simulink model "QuadModelv"  (R2022a)
settings: Solver=ode4  StartTime=0.0  StopTime=inf  FixedStep=0.001  RelTol=1e-3
PreLoadFcn:
  | filepath  = fileparts(get_param(bdroot, 'FileName'));
  | cd(filepath);
InitFcn:
  | Init
values from neighbouring files (symbols this model uses):
  ModelFailEnable = 0    [Init.m]
  ModelInit_RPM = 0    [Init.m]
  ModelParam_BattHoverMinutes = 18    [Init.m]
  ModelParam_BattHoverThr = 0.609    [Init.m]
  ModelParam_envAltitude = -50    [Init.m]
  ModelParam_GPSEphFinal = 0.3    [Init.m]
  ModelParam_GPSEpvFinal = 0.4    [Init.m]
  ModelParam_GPSFix3DFix = 3    [Init.m]
  ModelParam_GPSSatsVisible = 10    [Init.m]
  ModelParam_motorCr = 842.1    [Init.m]
  ModelParam_motorJm = 0.0001287    [Init.m]
  ModelParam_motorMinThr = 0.05    [Init.m]
  ModelParam_motorT = 0.0214    [Init.m]
  ModelParam_motorWb = 22.83    [Init.m]
  ModelParam_noiseGPSSampTime = 0.2    [Init.m]
  ModelParam_noisePowerOffGainAccel = 0.04    [Init.m]
  ModelParam_noisePowerOffGainAccelZ = 0.03    [Init.m]
  ModelParam_noisePowerOffGainGyro = 0.02    [Init.m]
  ModelParam_noisePowerOffGainGyroZ = 0.025    [Init.m]
  ModelParam_noisePowerOffGainMag = 0.02    [Init.m]
  ModelParam_noisePowerOffGainMagZ = 0.035    [Init.m]
  ModelParam_noisePowerOnGainAccel = 0.8    [Init.m]
  ModelParam_noisePowerOnGainAccelZ = 4.5    [Init.m]
  ModelParam_noisePowerOnGainGyro = 2    [Init.m]
  ModelParam_noisePowerOnGainGyroZ = 1    [Init.m]
  ModelParam_noisePowerOnGainMag = 0.025    [Init.m]
  ModelParam_noisePowerOnGainMagZ = 0.05    [Init.m]
  ModelParam_rotorCm = 2.783e-07    [Init.m]
  ModelParam_rotorCt = 1.681e-05    [Init.m]
  ModelParam_uavCCm = [0.0035 0.0039 0.0034]    [Init.m]
  ModelParam_uavCd = 0.055    [Init.m]
  ModelParam_uavDearo = 0.12    [Init.m]
  ModelParam_uavJ = [ModelParam_uavJxx,0,0;0,ModelParam_uavJyy,0;0,0,ModelParam_uavJzz]    [Init.m]
  ModelParam_uavMass = 1.515    [Init.m]
  ModelParam_uavMotNumbs = int8(4)    [Init.m]
  ModelParam_uavR = 0.225    [Init.m]
  ModelParam_uavType = int8(3)    [Init.m]
undefined symbols (not defined in the file or in its folder): d_i, Earth, h_i, ModelParam_GPSEpvInitial, ModelParam_GPSEpvTimeConstant, Newton, Raphson, WGS84
libraries: simulink x9, QuadModelLib x7, sharedtransform x3, aerolibtransform2 x2, sharedutil x2, aerolibutil x2, aerolibasang x2, shared6dof x1, aerolibatmos2 x1, aerolibconvert2 x1, aerolibobsolete x1
(part 1 of 3)
settings Model: Creator=Jinrui  LastModifiedBy=Tujinhu
settings SolverCC: AlgebraicLoopSolver=TrustRegion
settings DataIOCC: ReturnWorkspaceOutputs=off
settings OptimizationCC: ZeroExternalMemoryAtStartup=off  ZeroInternalMemoryAtStartup=off  EfficientTunableParamExpr=on
settings DebuggingCC: ParameterTunabilityLossMsg=error  UnconnectedInputMsg=warning  UnconnectedOutputMsg=warning  UnconnectedLineMsg=warning  SFMachineParentedDataDiag=warning  ArithmeticOperatorsInVariantConditions=warning
settings SFSimCC: SimUseLocalCustomCode=off  MATLABDynamicMemAlloc=off  CustomCodeUndefinedFunction=UseInterfaceOnly  SimTargetLang=C++
settings RTWCC: SystemTargetFile=ert.tlc  GenerateMakefile=off  PackageGeneratedCodeAndArtifacts=on  PackageName=MulticopterModel  TemplateMakefile=ert_default_tmf  RTWUseLocalCustomCode=off  TargetLang=C++  RTWCompilerOptimization=on  DLArmComputeVersion=19.05
settings CodeAppCC: ForceParamTrailComments=on  OperatorAnnotations=on  SimulinkDataObjDesc=on  SFDataObjDesc=on  MATLABFcnDesc=on  InsertBlockDesc=on  StateflowObjectComments=on  MATLABSourceComments=on
settings ERTTargetCC: TargetLangStandard=C++03 (ISO)  MultiwordLength=2048  GenerateSampleERTMain=on  CodeInterfacePackaging=C++ class  SupportContinuousTime=on  SupportVariableSizeSignals=on  MultiInstanceErrorCode=None  RootIOFormat=Structure reference  ERTCustomFileTemplate=example_file_process.tlc  ERTFilePackagingFormat=Compact
settings SimscapeCC: SimscapeNormalizeSystem=off

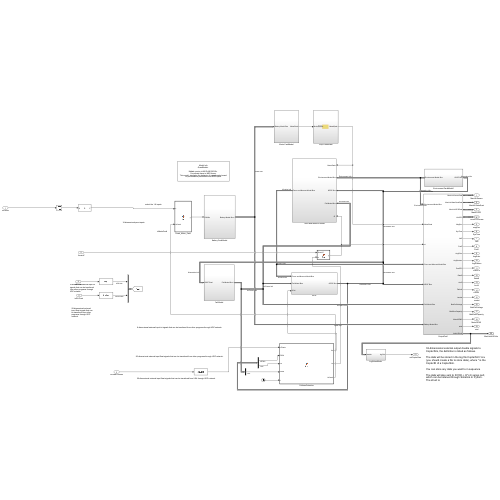
[thumbnail: Simulink's stored preview of the top-level diagram]
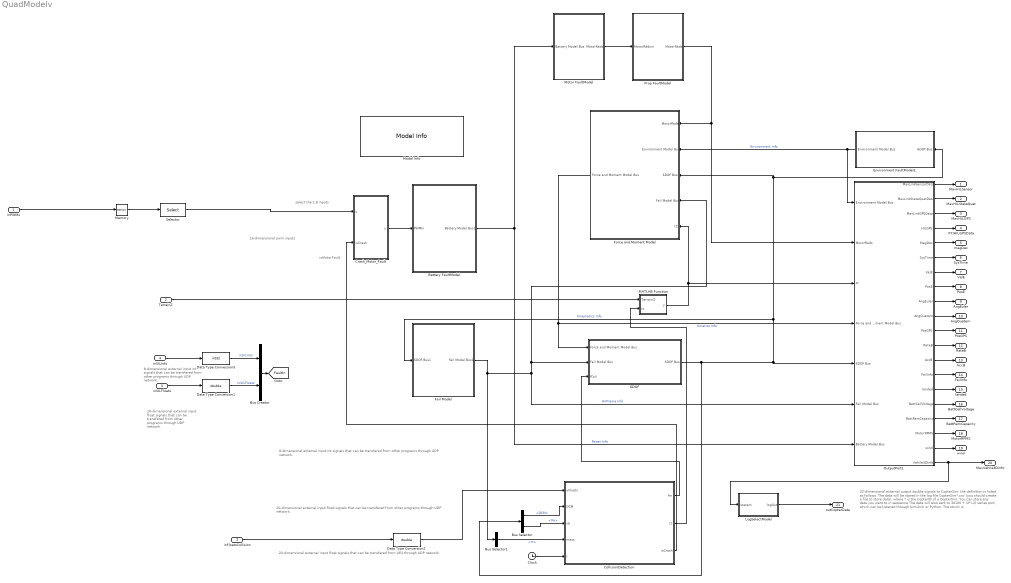
== system QuadModelv ==
  note: 16-dimensional pwm inputs
  note: 20-dimensional external input float signals that can be transfered from UE4 through UDP network.
  note: select the 1:8 inputs
  note: 8-dimensional external input int signals that can be transfered from other programs through UDP network.
  note: 20-dimensional external input float signals that can be transfered from other programs through UDP network.
  note: isMotorFault
  note: 20-dimensional external input float signals that can be transfered from other programs through UDP network.
  note: 8-dimensional external input int signals that can be transfered from other programs through UDP network.
  note: 32-dimensional external output double signals to CopterSim, the definition is listed as follows.
      |
      | The data will be stored in the log file CopterSim*.csv (you should create a file to store data), where * is the CopterID of a CopterSim.
      |
      | You can store any data you want to in sequence
      |
      | The data will also sent to 30100 + (2*i-2) series port, which can be listened through Simulink or Python. The struct is
  inPWMs : Inport  PortDimensions=8
  TerrainZ : Inport  Port=2  PortDimensions=1
  inFloatsCollision : Inport  Port=3  OutDataTypeStr=single  PortDimensions=20
  inSILInts : Inport  Port=4  OutDataTypeStr=int32  PortDimensions=8
  inSILFloats : Inport  Port=5  OutDataTypeStr=single  PortDimensions=20
  6DOF : Subsystem
  Battery FaultModel : Subsystem
  Bus Creator : BusCreator  Inputs=2
  Bus Selector : BusSelector  OutputSignals=DCM,Ve
  Bus Selector1 : BusSelector  OutputSignals=m
  Clock : Clock
  CollisionDetection : MATLAB Function  TreatAsAtomicUnit=on
  Crash_Motor_Fault : MATLAB Function  TreatAsAtomicUnit=on
  Data Type Conversion1 : DataTypeConversion  OutDataTypeStr=double  SaturateOnIntegerOverflow=off  RndMeth=Floor
  Data Type Conversion2 : DataTypeConversion  OutDataTypeStr=double  SaturateOnIntegerOverflow=off  RndMeth=Floor
  Data Type Conversion3 : DataTypeConversion  OutDataTypeStr=int32  SaturateOnIntegerOverflow=off  RndMeth=Floor
  Environment FaultModel1 : Subsystem
  Fail Model : Subsystem
  Force and Moment Model : Subsystem
  LogSelectModel : Subsystem
  MATLAB Function : MATLAB Function  TreatAsAtomicUnit=on
  Memory : Memory
  Model Info : simulink/Model-Wide Utilities/Model Info  Frame=on  DisplayStringWithTags=|  HorizontalTextAlignment=Center  LeftAlignmentValue=0.5
      | Model Info
      | %<ModelName> 
      | %<Description>   
      | Matlab version is MATLAB R2016b. 
      | Coordinate frame is NED frame.
      |  This model  simulates the behavior of a quadcopter based 
      | on performance parameters and RPM inputs
  Motor FaultModel : Subsystem
  OutputPort1 : Subsystem
  Prop FaultModel : Subsystem
  Selector : Selector  InputPortWidth=8  IndexOptions=Index vector (dialog)  Indices=[1:8]  OutputSizes=1
  MavHILSensor : Outport
  MavHILStateQuat : Outport  Port=2  OutDataTypeStr=Bus: MavLinkStateQuat  VectorParamsAs1DForOutWhenUnconnected=off
  MavHILGPS : Outport  Port=3
  PXIHILGPSData : Outport  Port=4  OutDataTypeStr=Bus: HILGPS  VectorParamsAs1DForOutWhenUnconnected=off
  magDec : Outport  Port=5  VectorParamsAs1DForOutWhenUnconnected=off
  SysTime : Outport  Port=6  VectorParamsAs1DForOutWhenUnconnected=off
  VelE : Outport  Port=7  VectorParamsAs1DForOutWhenUnconnected=off
  PosE : Outport  Port=8  VectorParamsAs1DForOutWhenUnconnected=off
  AngEuler : Outport  Port=9  VectorParamsAs1DForOutWhenUnconnected=off
  AngQuatern : Outport  Port=10  VectorParamsAs1DForOutWhenUnconnected=off
  PosGPS : Outport  Port=11  VectorParamsAs1DForOutWhenUnconnected=off
  RateB : Outport  Port=12  VectorParamsAs1DForOutWhenUnconnected=off
  AccB : Outport  Port=13  VectorParamsAs1DForOutWhenUnconnected=off
  FailInfo : Outport  Port=14  VectorParamsAs1DForOutWhenUnconnected=off
  landed : Outport  Port=15  VectorParamsAs1DForOutWhenUnconnected=off
  BattCellVoltage : Outport  Port=16  VectorParamsAs1DForOutWhenUnconnected=off
  BattRemCapacity : Outport  Port=17  VectorParamsAs1DForOutWhenUnconnected=off
  MotorRPMS : Outport  Port=18  VectorParamsAs1DForOutWhenUnconnected=off
  wind : Outport  Port=19  VectorParamsAs1DForOutWhenUnconnected=off
  MavVehile3DInfo : Outport  Port=20  OutDataTypeStr=Bus: MavVehileInfo  VectorParamsAs1DForOutWhenUnconnected=off
  outCopterData : Outport  Port=21  OutDataTypeStr=double  PortDimensions=32  VectorParamsAs1DForOutWhenUnconnected=off
  tag scope: FaultIn=global
  wires:
  OutputPort1/14(FailInfo) -> FailInfo/1
  OutputPort1/9(AngEuler) -> AngEuler/1
  OutputPort1/17(BattRemCapacity) -> BattRemCapacity/1
  Memory/1 -> Selector/1
  OutputPort1/1(MavLinkSensorData) -> MavHILSensor/1
  Force and Moment Model/1(Force and Moment Model Bus) -> 6DOF/1(Force and Moment Model Bus), OutputPort1/4(Force and Moment Model Bus)  "Kinetics Info"
  Battery FaultModel/1(Battery Model Bus1) -> Motor FaultModel/1(Battery Model Bus), OutputPort1/7(Battery Model Bus)  "Power Info"
  Fail Model/1(Fail Model Bus1) -> Bus Selector1/1, Force and Moment Model/4(Fail Model Bus), 6DOF/2(Fail Model Bus), OutputPort1/6(Fail Model Bus)  "AirFrame Info"
  Bus Selector1/1 -> CollisionDetection/4(mass)  "<m>"
  OutputPort1/15(landed) -> landed/1
  TerrainZ/1 -> MATLAB Function/1(TerrainZ)
  OutputPort1/8(PosE) -> PosE/1
  OutputPort1/19(wind) -> wind/1
  Environment FaultModel1/1(Environment Model Bus) -> OutputPort1/1(Environment Model Bus), Force and Moment Model/2(Environment Model Bus)  "Environment Info"
  inFloatsCollision/1 -> Data Type Conversion2/1
  Bus Selector/1 -> CollisionDetection/2(DCM)  "<DCM>"
  inPWMs/1 -> Memory/1
  MATLAB Function/1(y) -> Force and Moment Model/5("tZ "), OutputPort1/3(zt)
  CollisionDetection/2(tz) -> MATLAB Function/2(tz)
  Prop FaultModel/1(MotorRads) -> OutputPort1/2(MotorRads), Force and Moment Model/1(MotorRads)
  OutputPort1/10(AngQuatern) -> AngQuatern/1
  OutputPort1/7(VelE) -> VelE/1
  OutputPort1/13(AccB) -> AccB/1
  6DOF/1(6DOF Bus) -> Bus Selector/1, Fail Model/1(6DOF Bus1), Environment FaultModel1/1(6DOF Bus), Force and Moment Model/3(6DOF Bus), OutputPort1/5(6DOF Bus)  "Kinematics Info"
  OutputPort1/12(RateB) -> RateB/1
  OutputPort1/5(MagDec) -> magDec/1
  CollisionDetection/1(fm) -> 6DOF/3(fColi)
  OutputPort1/18(MotorRPMS) -> MotorRPMS/1
  OutputPort1/16(BattCellVoltage) -> BattCellVoltage/1
  OutputPort1/20(Vehile3DInfo) -> LogSelectModel/1(stateIn), MavVehile3DInfo/1
  CollisionDetection/3(isCrash) -> Crash_Motor_Fault/2(isCrash)
  Bus Selector/2 -> CollisionDetection/3(ve)  "<Ve>"
  OutputPort1/2(MavLinkStateQuatData) -> MavHILStateQuat/1
  OutputPort1/3(MavLinkGPSData) -> MavHILGPS/1
  Data Type Conversion2/1 -> CollisionDetection/1(uFloats)
  OutputPort1/6(SysTime) -> SysTime/1
  OutputPort1/4(HILGPS) -> PXIHILGPSData/1
  OutputPort1/11(PosGPS) -> PosGPS/1
  Clock/1 -> CollisionDetection/5(t)
  Data Type Conversion3/1 -> Bus Creator/1  "inSILInts"
  Data Type Conversion1/1 -> Bus Creator/2  "inSILFloats"
  Bus Creator/1 -> [FaultIn]
  LogSelectModel/1(logOut) -> outCopterData/1
  Motor FaultModel/1(MotorRads) -> Prop FaultModel/1(MotorRadsin)
  Crash_Motor_Fault/1(y) -> Battery FaultModel/1(PWMIn)
  Selector/1 -> Crash_Motor_Fault/1(u)
  inSILInts/1 -> Data Type Conversion3/1
  inSILFloats/1 -> Data Type Conversion1/1

== system QuadModelv/6DOF ==
  Force and Moment Model Bus : Inport
  Fail Model Bus : Inport  Port=2
  fColi : Inport  Port=3
  Bus Creator : BusCreator  Inputs=8
  Bus Selector : BusSelector  OutputSignals=dM,m,J
  Bus Selector1 : BusSelector  OutputSignals=Fb,Mb
  Constant_dI/dt : Constant  Value=zeros(3,3)
  Custom Variable Mass 6DOF (Quaternion) : shared6dof/6DOF (Euler Angles)  units=Metric (MKS)  mtype=Custom Variable  rep=Quaternion  xme_0=ModelInit_PosE  Vm_0=ModelInit_VelB  eul_0=ModelInit_AngEuler  pm_0=ModelInit_RateB  mass_0=1.0  mass_e=0.5  mass_f=2.0  inertia=eye(3)  inertia_e=eye(3)  inertia_f=2*eye(3)  k_quat=1.0  vre_flag=off  abi_flag=off  aMode=aMode  xme_statename=''  Vm_statename=''  eul_statename=''  quat_statename=''  pm_statename=''  mass_statename=''
      settings: SourceProductBaseCode=AE,PW,DR,MT,VE
  Demux : Demux  Outputs=2
  Sum : Sum  Inputs=+++
  Sum1 : Sum  Inputs=++|
  6DOF Bus : Outport  VectorParamsAs1DForOutWhenUnconnected=off
  wires:
  Bus Selector1/1 -> Sum1/2  "<Fb>"
  Bus Selector/2 -> Custom Variable Mass 6DOF (Quaternion)/3  "<m>"
  Custom Variable Mass 6DOF (Quaternion)/8 -> Bus Creator/8  "AccB"
  Sum/1 -> Custom Variable Mass 6DOF (Quaternion)/2
  Constant_dI/dt/1 -> Custom Variable Mass 6DOF (Quaternion)/4
  Custom Variable Mass 6DOF (Quaternion)/5 -> Bus Creator/5  "Vb"
  Custom Variable Mass 6DOF (Quaternion)/6 -> Bus Creator/6  "wb"
  Custom Variable Mass 6DOF (Quaternion)/1 -> Bus Creator/1  "Ve"
  Custom Variable Mass 6DOF (Quaternion)/4 -> Bus Creator/4  "DCM"
  Custom Variable Mass 6DOF (Quaternion)/2 -> Bus Creator/2  "Xe"
  Custom Variable Mass 6DOF (Quaternion)/3 -> Bus Creator/3  "Eular(rad)"
  Custom Variable Mass 6DOF (Quaternion)/7 -> Bus Creator/7  "dwb/dt"
  Bus Selector/3 -> Custom Variable Mass 6DOF (Quaternion)/5  "<J>"
  Bus Selector/1 -> Sum/2  "<dM>"
  Bus Selector1/2 -> Sum/1  "<Mb>"
  Fail Model Bus/1 -> Bus Selector/1
  Force and Moment Model Bus/1 -> Bus Selector1/1
  Bus Creator/1 -> 6DOF Bus/1
  Sum1/1 -> Custom Variable Mass 6DOF (Quaternion)/1
  Demux/1 -> Sum1/1
  fColi/1 -> Demux/1
  Demux/2 -> Sum/3

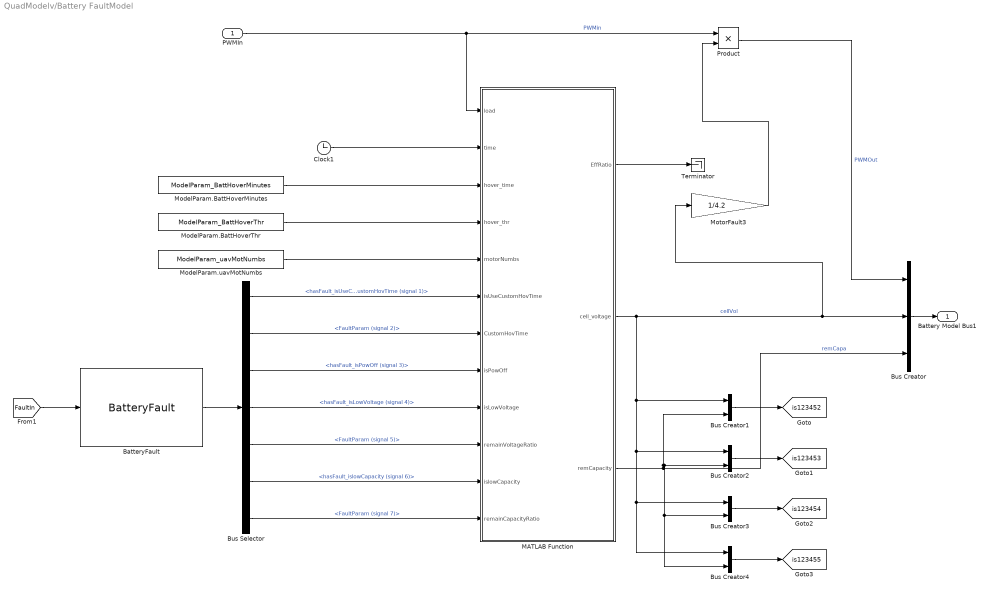
== system QuadModelv/Battery FaultModel ==
  PWMIn : Inport
  BatteryFault : QuadModelLib/BatteryFault  FaultParamStruct=BatteryFault
  Bus Creator : BusCreator  Inputs=3
  Bus Creator{1..4} (4 alike) : BusCreator  Inputs=2
  Bus Selector : BusSelector  OutputSignals=hasFault_isUseCustomHovTime (signal 1),FaultParam (signal 2),hasFault_isPowOff (signal 3),hasFault_isLowVoltage (signal 4),FaultParam (signal 5),hasFault_islowCapacity (signal 6),FaultParam (signal 7)
  Clock1 : Clock
  MATLAB Function : MATLAB Function  TreatAsAtomicUnit=on  SystemSampleTime=0.01
  ModelParam.BattHoverMinutes : Constant  Value=ModelParam_BattHoverMinutes
  ModelParam.BattHoverThr : Constant  Value=ModelParam_BattHoverThr
  ModelParam.uavMotNumbs : Constant  Value=ModelParam_uavMotNumbs
  MotorFault3 : Gain  Gain=1/4.2
  Product : Product
  Terminator : Terminator
  Battery Model Bus1 : Outport  VectorParamsAs1DForOutWhenUnconnected=off
  tag scope: is123452=global, is123453=global, is123454=global, is123455=global
  wires:
  Bus Selector/7 -> MATLAB Function/12(remainCapacityRatio)  "<FaultParam (signal 7)>"
  Bus Creator4/1 -> [is123455]
  MATLAB Function/2(cell_voltage) -> Bus Creator4/1, Bus Creator3/1, Bus Creator2/1, Bus Creator1/1, MotorFault3/1, Bus Creator/2  "cellVol"
  MATLAB Function/3(remCapacity) -> Bus Creator1/2, Bus Creator4/2, Bus Creator3/2, Bus Creator2/2, Bus Creator/3  "remCapa"
  Bus Selector/2 -> MATLAB Function/7(CustomHovTime)  "<FaultParam (signal 2)>"
  ModelParam.uavMotNumbs/1 -> MATLAB Function/5(motorNumbs)
  Bus Creator/1 -> Battery Model Bus1/1
  Bus Creator1/1 -> [is123452]
  Bus Creator2/1 -> [is123453]
  ModelParam.BattHoverThr/1 -> MATLAB Function/4(hover_thr)
  Bus Creator3/1 -> [is123454]
  MATLAB Function/1(EffRatio) -> Terminator/1
  ModelParam.BattHoverMinutes/1 -> MATLAB Function/3(hover_time)
  Product/1 -> Bus Creator/1  "PWMOut"
  PWMIn/1 -> MATLAB Function/1(load), Product/1  "PWMin"
  Bus Selector/6 -> MATLAB Function/11(islowCapacity)  "<hasFault_islowCapacity (signal 6)>"
  Bus Selector/3 -> MATLAB Function/8(isPowOff)  "<hasFault_isPowOff (signal 3)>"
  Clock1/1 -> MATLAB Function/2(time)
  BatteryFault/1 -> Bus Selector/1
  Bus Selector/4 -> MATLAB Function/9(isLowVoltage)  "<hasFault_isLowVoltage (signal 4)>"
  [FaultIn] -> BatteryFault/1
  MotorFault3/1 -> Product/2
  Bus Selector/1 -> MATLAB Function/6(isUseCustomHovTime)  "<hasFault_isUseCustomHovTime (signal 1)>"
  Bus Selector/5 -> MATLAB Function/10(remainVoltageRatio)  "<FaultParam (signal 5)>"

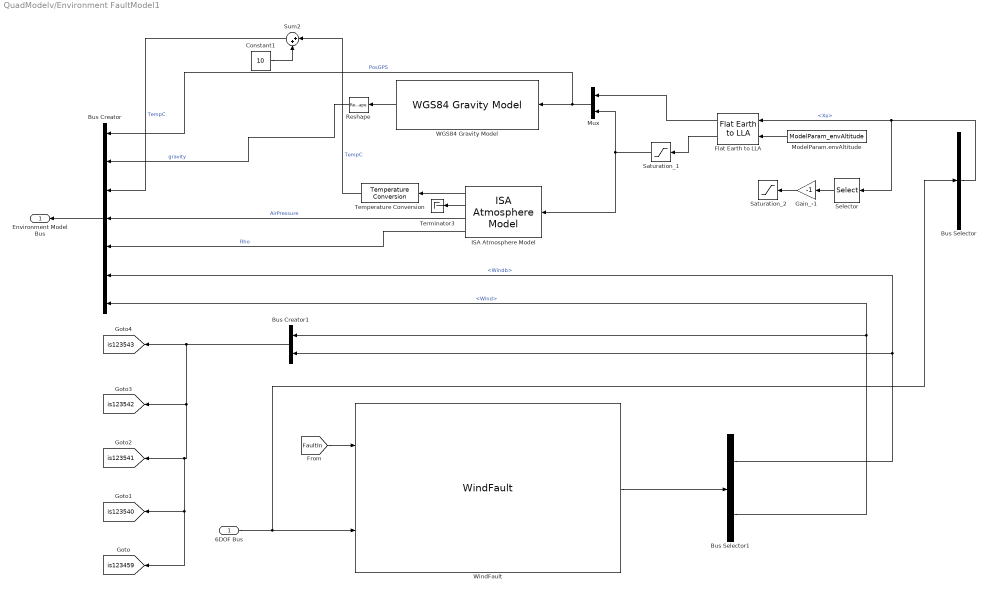
== system QuadModelv/Environment FaultModel1 ==
  6DOF Bus : Inport
  Bus Creator : BusCreator  Inputs=7
  Bus Creator1 : BusCreator  Inputs=2
  Bus Selector : BusSelector  OutputSignals=Xe
  Bus Selector1 : BusSelector  OutputSignals=Windb,Wind
  Constant1 : Constant  Value=10
  Flat Earth to LLA : aerolibtransform2/Flat Earth to LLA  units=Metric (MKS)  ptype=Earth (WGS84)  F=1/298.257223563  R=6378137  refPosPort=off  LL0=ModelParam_GPSLatLong  psi=0
  Gain_-1 : Gain  Gain=-1
  ISA Atmosphere Model : aerolibatmos2/ISA Atmosphere Model  custom=off  g=9.80665  gamma=1.4  R=287.0531  L=0.0065  h_trop=11000  h_strat=20000  rho0=1.225  P0=101325  T0=288.15  h0=0
  ModelParam.envAltitude : Constant  Value=ModelParam_envAltitude
  Mux : Mux  Inputs=2
  Reshape : Reshape
  Saturation_1 : Saturate  UpperLimit=100000  LowerLimit=0
  Saturation_2 : Saturate  UpperLimit=10000  LowerLimit=0
  Selector : Selector  InputPortWidth=3  IndexOptions=Index vector (dialog)  Indices=[3]  OutputSizes=1
  Sum2 : Sum  Inputs=|++
  Temperature Conversion : aerolibconvert2/Temperature Conversion  IU=K  OU=C
      settings: SourceProductBaseCode=AE
  Terminator3 : Terminator
  "WGS84 Gravity Model " : aerolibobsolete/WGS84 Gravity Model   model=WGS84 Taylor Series  units=Metric (MKS)  no_atmos=on  precessing=on  jd_loc=off  month=October  day=10  year=2004  no_centrifugal=on  action=Warning
      settings: SourceProductBaseCode=AE
  WindFault : QuadModelLib/WindFault  FaultParamStruct=WindFault  ComParamVect=FaultParamAPI
  Environment Model Bus : Outport  VectorParamsAs1DForOutWhenUnconnected=off
  tag scope: is123459=global, is123540=global, is123541=global, is123542=global, is123543=global
  wires:
  ISA Atmosphere Model/2 -> Terminator3/1
  Bus Selector/1 -> Selector/1, Flat Earth to LLA/1  "<Xe>"
  Flat Earth to LLA/1 -> Mux/1
  Mux/1 -> Bus Creator/1, "WGS84 Gravity Model "/1  "PosGPS"
  ISA Atmosphere Model/3 -> Bus Creator/4  "AirPressure"
  Selector/1 -> Gain_-1/1
  Sum2/1 -> Bus Creator/3  "TempC"
  Temperature Conversion/1 -> Sum2/1  "TempC"
  ModelParam.envAltitude/1 -> Flat Earth to LLA/2
  Constant1/1 -> Sum2/2
  Reshape/1 -> Bus Creator/2  "gravity"
  "WGS84 Gravity Model "/1 -> Reshape/1
  Gain_-1/1 -> Saturation_2/1
  6DOF Bus/1 -> WindFault/2, Bus Selector/1
  Bus Creator/1 -> Environment Model Bus/1
  Bus Selector1/2 -> Bus Creator/7, Bus Creator1/1  "<Wind>"
  Bus Creator1/1 -> [is123459], [is123540], [is123541], [is123542], [is123543]
  ISA Atmosphere Model/1 -> Temperature Conversion/1
  Saturation_1/1 -> Mux/2, ISA Atmosphere Model/1
  Bus Selector1/1 -> Bus Creator/6, Bus Creator1/2  "<Windb>"
  [FaultIn] -> WindFault/1
  ISA Atmosphere Model/4 -> Bus Creator/5  "Rho"
  Flat Earth to LLA/2 -> Saturation_1/1
  WindFault/1 -> Bus Selector1/1

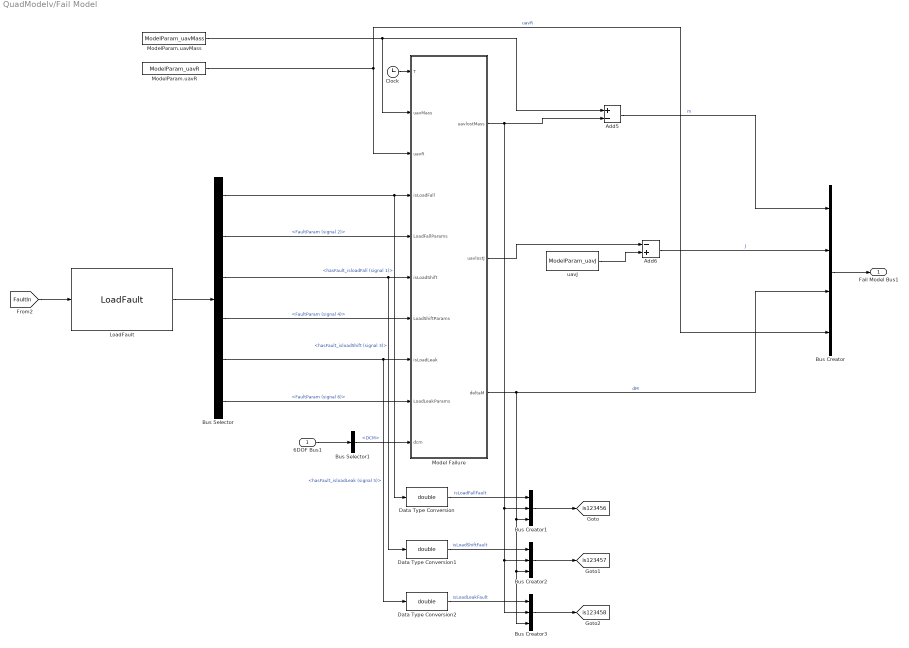
== system QuadModelv/Fail Model ==
  6DOF Bus1 : Inport
  Add5 : Sum  Inputs=+-
  Add6 : Sum  Inputs=-+
  Bus Creator : BusCreator  Inputs=4
  Bus Creator1 : BusCreator  Inputs=3
  Bus Creator2 : BusCreator  Inputs=3
  Bus Creator3 : BusCreator  Inputs=3
  Bus Selector : BusSelector  OutputSignals=hasFault_isloadFall (signal 1),FaultParam (signal 2),hasFault_isloadShift (signal 3),FaultParam (signal 4),hasFault_isloadLeak (signal 5),FaultParam (signal 6)
  Bus Selector1 : BusSelector  OutputSignals=DCM
  Clock : Clock
  Data Type Conversion : DataTypeConversion  OutDataTypeStr=double  SaturateOnIntegerOverflow=off  RndMeth=Floor
  Data Type Conversion1 : DataTypeConversion  OutDataTypeStr=double  SaturateOnIntegerOverflow=off  RndMeth=Floor
  Data Type Conversion2 : DataTypeConversion  OutDataTypeStr=double  SaturateOnIntegerOverflow=off  RndMeth=Floor
  LoadFault : QuadModelLib/LoadFault  FaultParamStruct=LoadFault
  Model Failure : MATLAB Function  TreatAsAtomicUnit=on
  ModelParam.uavMass : Constant  Value=ModelParam_uavMass
  ModelParam.uavR : Constant  Value=ModelParam_uavR
  uavJ : Constant  Value=ModelParam_uavJ
  Fail Model Bus1 : Outport  VectorParamsAs1DForOutWhenUnconnected=off
  tag scope: is123456=global, is123457=global, is123458=global
  wires:
  Bus Selector/3 -> Data Type Conversion1/1, Model Failure/6(isLoadShift)  "<hasFault_isloadShift (signal 3)>"
  Data Type Conversion2/1 -> Bus Creator3/1  "isLoadLeakFault"
  Model Failure/3(deltaM) -> Bus Creator1/3, Bus Creator3/3, Bus Creator2/3, Bus Creator/3  "dM"
  Data Type Conversion/1 -> Bus Creator1/1  "isLoadFallFault"
  Bus Creator2/1 -> [is123457]
  Bus Creator1/1 -> [is123456]
  Data Type Conversion1/1 -> Bus Creator2/1  "isLoadShiftFault"
  Bus Creator/1 -> Fail Model Bus1/1
  Bus Selector/6 -> Model Failure/9(LoadLeakParams)  "<FaultParam (signal 6)>"
  Bus Creator3/1 -> [is123458]
  Bus Selector1/1 -> Model Failure/10(dcm)  "<DCM>"
  uavJ/1 -> Add6/2
  Model Failure/2(uavlostJ) -> Add6/1
  ModelParam.uavR/1 -> Model Failure/3(uavR), Bus Creator/4  "uavR"
  Bus Selector/1 -> Model Failure/4(isLoadFall), Data Type Conversion/1  "<hasFault_isloadFall (signal 1)>"
  Add6/1 -> Bus Creator/2  "J"
  6DOF Bus1/1 -> Bus Selector1/1
  Bus Selector/2 -> Model Failure/5(LoadFallParams)  "<FaultParam (signal 2)>"
  Add5/1 -> Bus Creator/1  "m"
  Bus Selector/4 -> Model Failure/7(LoadShiftParams)  "<FaultParam (signal 4)>"
  Bus Selector/5 -> Data Type Conversion2/1, Model Failure/8(isLoadLeak)  "<hasFault_isloadLeak (signal 5)>"
  Clock/1 -> Model Failure/1(T)
  Model Failure/1(uavlostMass) -> Bus Creator1/2, Bus Creator3/2, Bus Creator2/2, Add5/2
  [FaultIn] -> LoadFault/1
  LoadFault/1 -> Bus Selector/1
  ModelParam.uavMass/1 -> Model Failure/2(uavMass), Add5/1

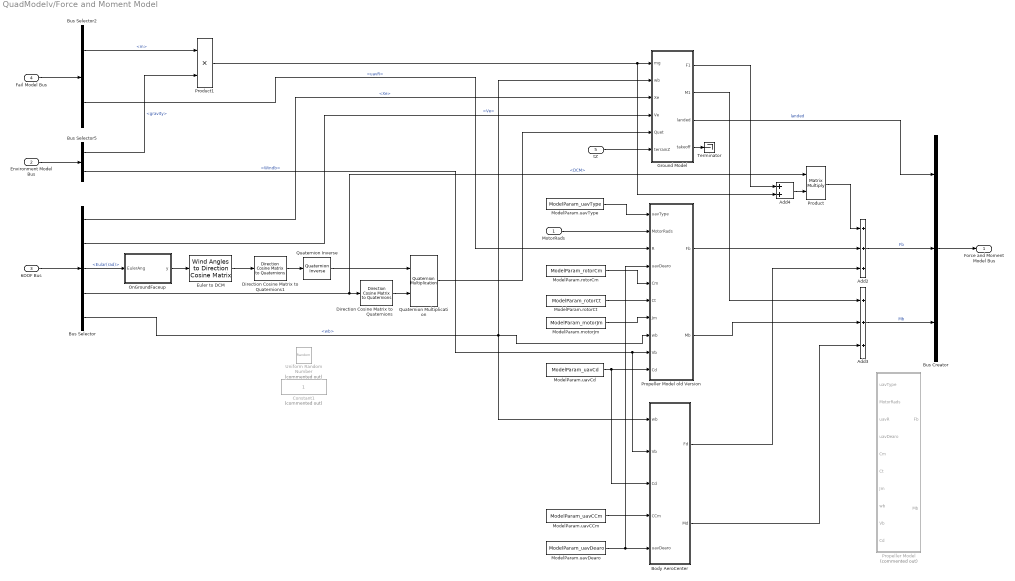
== system QuadModelv/Force and Moment Model ==
  MotorRads : Inport
  Environment Model Bus : Inport  Port=2
  6DOF Bus : Inport  Port=3
  Fail Model Bus : Inport  Port=4
  "tZ " : Inport  Port=5
  Add2 : Sum  Inputs=+++
  Add3 : Sum  Inputs=+++
  Add4 : Sum
  Body AeroCenter : MATLAB Function  TreatAsAtomicUnit=on
  Bus Creator : BusCreator  Inputs=3
  Bus Selector : BusSelector  OutputSignals=Xe,Ve,Eular(rad),DCM,wb
  Bus Selector2 : BusSelector  OutputSignals=m,uavR
  Bus Selector5 : BusSelector  OutputSignals=gravity,Windb
  Constant1 : Constant  Commented=on
  Direction Cosine Matrix to Quaternions : sharedtransform/Direction Cosine Matrix  to Quaternions  aMode=aMode  action=None  tolerance=eps(2)
      settings: SourceProductBaseCode=AE,PW,DR,MT,VE
  Direction Cosine Matrix to Quaternions1 : sharedtransform/Direction Cosine Matrix  to Quaternions  aMode=aMode  action=None  tolerance=eps(2)
      settings: SourceProductBaseCode=AE,PW,DR,MT,VE
  Euler to DCM : aerolibtransform2/Wind Angles to  Direction Cosine Matrix
      settings: SourceProductBaseCode=AE
  Ground Model : MATLAB Function  TreatAsAtomicUnit=on
  ModelParam.motorJm : Constant  Value=ModelParam_motorJm
  ModelParam.rotorCm : Constant  Value=ModelParam_rotorCm
  ModelParam.rotorCt : Constant  Value=ModelParam_rotorCt
  ModelParam.uavCCm : Constant  Value=ModelParam_uavCCm
  ModelParam.uavCd : Constant  Value=ModelParam_uavCd
  ModelParam.uavDearo : Constant  Value=ModelParam_uavDearo
  ModelParam.uavType : Constant  Value=ModelParam_uavType
  OnGroundFaceup : MATLAB Function  TreatAsAtomicUnit=on
  Product : Product  Multiplication=Matrix(*)
  Product1 : Product
  Propeller Model : Subsystem  Commented=on  TreatAsAtomicUnit=on
  Propeller Model old Version : MATLAB Function  TreatAsAtomicUnit=on
  Quaternion Inverse : aerolibutil/Quaternion Inverse
  Quaternion Multiplication : aerolibutil/Quaternion Multiplication
  Terminator : Terminator
  Uniform Random Number : UniformRandomNumber  Commented=on  Minimum=[-1,-1,-1]  Maximum=[1,1,1]  Seed=[145787,351545,2864]  SampleTime=0.05
  Force and Moment Model Bus : Outport  VectorParamsAs1DForOutWhenUnconnected=off
  wires:
  Body AeroCenter/2(Md) -> Add3/3
  Body AeroCenter/1(Fd) -> Add2/3
  Propeller Model old Version/2(Mb) -> Add3/2
  Propeller Model old Version/1(Fb) -> Add2/2
  Ground Model/4(takeoff) -> Terminator/1
  Ground Model/3(landed) -> Bus Creator/1  "landed"
  "tZ "/1 -> Ground Model/6(terrainZ)
  Add3/1 -> Bus Creator/3  "Mb"
  Add2/1 -> Bus Creator/2  "Fb"
  ModelParam.uavType/1 -> Propeller Model old Version/1(uavType)
  Quaternion Multiplication/1 -> Ground Model/5(Quet)
  Quaternion Inverse/1 -> Quaternion Multiplication/1
  Direction Cosine Matrix to Quaternions1/1 -> Quaternion Inverse/1
  Euler to DCM/1 -> Direction Cosine Matrix to Quaternions1/1
  OnGroundFaceup/1(y) -> Euler to DCM/1
  Direction Cosine Matrix to Quaternions/1 -> Quaternion Multiplication/2
  ModelParam.rotorCt/1 -> Propeller Model old Version/6(Ct)
  Product/1 -> Add2/1
  Ground Model/1(F1) -> Add4/1
  Add4/1 -> Product/2
  Product1/1 -> Ground Model/1(mg), Add4/2
  Ground Model/2(M1) -> Add3/1
  Bus Selector/4 -> Direction Cosine Matrix to Quaternions/1, Product/1  "<DCM>"
  ModelParam.uavCd/1 -> Body AeroCenter/3(Cd), Propeller Model old Version/10(Cd)
  ModelParam.motorJm/1 -> Propeller Model old Version/7(Jm)
  ModelParam.rotorCm/1 -> Propeller Model old Version/5(Cm)
  MotorRads/1 -> Propeller Model old Version/2(MotorRads)
  Bus Selector/5 -> Ground Model/2(wb), Propeller Model old Version/8(wb), Body AeroCenter/1(wb)  "<wb>"
  ModelParam.uavCCm/1 -> Body AeroCenter/4(CCm)
  Bus Creator/1 -> Force and Moment Model Bus/1
  6DOF Bus/1 -> Bus Selector/1
  Bus Selector/2 -> Ground Model/4(Ve)  "<Ve>"
  Bus Selector/1 -> Ground Model/3(Xe)  "<Xe>"
  Bus Selector/3 -> OnGroundFaceup/1(EulerAng)  "<Eular(rad)>"
  Bus Selector2/1 -> Product1/1  "<m>"
  Bus Selector5/1 -> Product1/2  "<gravity>"
  Fail Model Bus/1 -> Bus Selector2/1
  Environment Model Bus/1 -> Bus Selector5/1
  Bus Selector2/2 -> Propeller Model old Version/3(R)  "<uavR>"
  Bus Selector5/2 -> Body AeroCenter/2(Vb), Propeller Model old Version/9(Vb)  "<Windb>"
  ModelParam.uavDearo/1 -> Propeller Model old Version/4(uavDearo), Body AeroCenter/5(uavDearo)

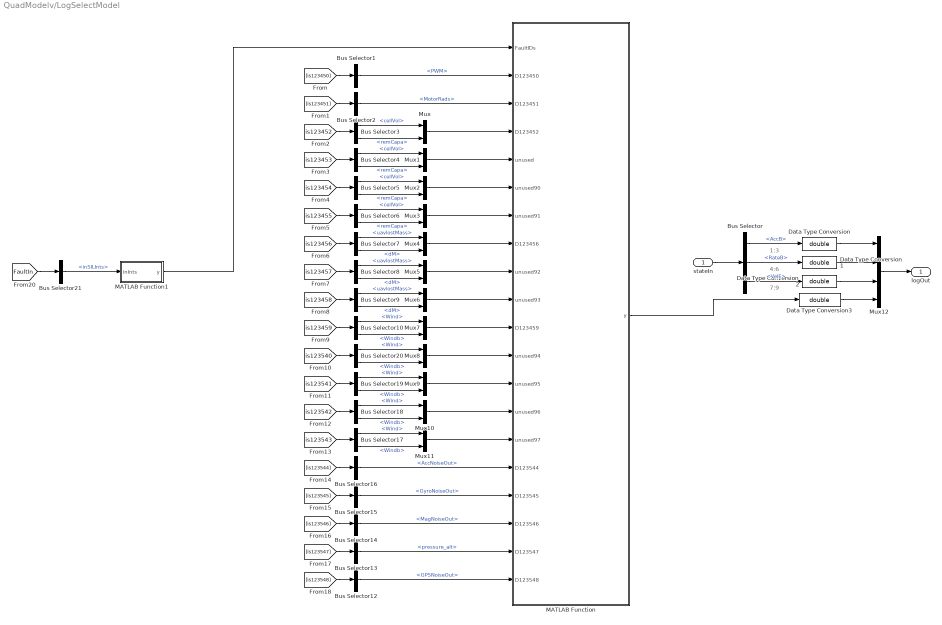
== system QuadModelv/LogSelectModel ==
  note: 1:3
  note: 4:6
  note: 7:9
  stateIn : Inport
  Bus Selector : BusSelector  OutputSignals=AccB,RateB,VelE
  Bus Selector1 : BusSelector  OutputSignals=PWM
  Bus Selector{10,17..20} (5 alike) : BusSelector  OutputSignals=Wind,Windb
  Bus Selector12 : BusSelector  OutputSignals=GPSNoiseOut
  Bus Selector13 : BusSelector  OutputSignals=pressure_alt
  Bus Selector14 : BusSelector  OutputSignals=MagNoiseOut
  Bus Selector15 : BusSelector  OutputSignals=GyroNoiseOut
  Bus Selector16 : BusSelector  OutputSignals=AccNoiseOut
  Bus Selector2 : BusSelector  OutputSignals=MotorRads
  Bus Selector21 : BusSelector  OutputSignals=inSILInts
  Bus Selector{3..6} (4 alike) : BusSelector  OutputSignals=cellVol,remCapa
  Bus Selector7 : BusSelector  OutputSignals=uavlostMass,dM
  Bus Selector8 : BusSelector  OutputSignals=uavlostMass,dM
  Bus Selector9 : BusSelector  OutputSignals=uavlostMass,dM
  Data Type Conversion{,1..3} (4 alike) : DataTypeConversion  OutDataTypeStr=double  SaturateOnIntegerOverflow=off  RndMeth=Floor
  MATLAB Function : MATLAB Function  TreatAsAtomicUnit=on
  MATLAB Function1 : MATLAB Function  TreatAsAtomicUnit=on
  Mux{,1..11} (12 alike) : Mux  Inputs=2
  Mux12 : Mux
  logOut : Outport
  wires:
  stateIn/1 -> Bus Selector/1
  Bus Selector/1 -> Data Type Conversion/1  "<AccB>"
  Bus Selector/2 -> Data Type Conversion1/1  "<RateB>"
  Bus Selector/3 -> Data Type Conversion2/1  "<VelE>"
  [FaultIn] -> Bus Selector21/1
  [is123452] -> Bus Selector3/1
  [is123542] -> Bus Selector18/1
  [is123541] -> Bus Selector19/1
  [is123459] -> Bus Selector10/1
  [is123546] -> Bus Selector14/1
  [is123451] -> Bus Selector2/1
  [is123548] -> Bus Selector12/1
  [is123454] -> Bus Selector5/1
  [is123544] -> Bus Selector16/1
  [is123547] -> Bus Selector13/1
  [is123453] -> Bus Selector4/1
  [is123458] -> Bus Selector9/1
  [is123540] -> Bus Selector20/1
  [is123543] -> Bus Selector17/1
  [is123545] -> Bus Selector15/1
  [is123455] -> Bus Selector6/1
  [is123450] -> Bus Selector1/1
  [is123456] -> Bus Selector7/1
  [is123457] -> Bus Selector8/1
  Bus Selector1/1 -> MATLAB Function/2(D123450)  "<PWM>"
  Bus Selector2/1 -> MATLAB Function/3(D123451)  "<MotorRads>"
  Bus Selector3/1 -> Mux/1  "<cellVol>"
  Bus Selector3/2 -> Mux/2  "<remCapa>"
  Mux/1 -> MATLAB Function/4(D123452)
  Bus Selector4/1 -> Mux1/1  "<cellVol>"
  Bus Selector4/2 -> Mux1/2  "<remCapa>"
  Bus Selector5/1 -> Mux2/1  "<cellVol>"
  Bus Selector5/2 -> Mux2/2  "<remCapa>"
  Mux2/1 -> MATLAB Function/6(unused90)
  Bus Selector6/1 -> Mux3/1  "<cellVol>"
  Bus Selector6/2 -> Mux3/2  "<remCapa>"
  Mux3/1 -> MATLAB Function/7(unused91)
  Bus Selector7/1 -> Mux4/1  "<uavlostMass>"
  Mux4/1 -> MATLAB Function/8(D123456)
  Bus Selector8/1 -> Mux5/1  "<uavlostMass>"
  Mux5/1 -> MATLAB Function/9(unused92)
  Bus Selector9/1 -> Mux6/1  "<uavlostMass>"
  Mux6/1 -> MATLAB Function/10(unused93)
  Bus Selector10/1 -> Mux7/1  "<Wind>"
  Bus Selector10/2 -> Mux7/2  "<Windb>"
  Mux7/1 -> MATLAB Function/11(D123459)
  Bus Selector20/1 -> Mux8/1  "<Wind>"
  Bus Selector20/2 -> Mux8/2  "<Windb>"
  Mux8/1 -> MATLAB Function/12(unused94)
  Bus Selector19/1 -> Mux9/1  "<Wind>"
  Bus Selector19/2 -> Mux9/2  "<Windb>"
  Mux9/1 -> MATLAB Function/13(unused95)
  Bus Selector18/1 -> Mux10/1  "<Wind>"
  Bus Selector18/2 -> Mux10/2  "<Windb>"
  Mux10/1 -> MATLAB Function/14(unused96)
  Bus Selector17/1 -> Mux11/1  "<Wind>"
  Bus Selector17/2 -> Mux11/2  "<Windb>"
  Mux11/1 -> MATLAB Function/15(unused97)
  Bus Selector16/1 -> MATLAB Function/16(D123544)  "<AccNoiseOut>"
  Bus Selector15/1 -> MATLAB Function/17(D123545)  "<GyroNoiseOut>"
  Bus Selector14/1 -> MATLAB Function/18(D123546)  "<MagNoiseOut>"
  Bus Selector13/1 -> MATLAB Function/19(D123547)  "<pressure_alt>"
  Bus Selector12/1 -> MATLAB Function/20(D123548)  "<GPSNoiseOut>"
  Bus Selector7/2 -> Mux4/2  "<dM>"
  Bus Selector8/2 -> Mux5/2  "<dM>"
  Bus Selector9/2 -> Mux6/2  "<dM>"
  Bus Selector21/1 -> MATLAB Function1/1(inInts)  "<inSILInts>"
  MATLAB Function1/1(y) -> MATLAB Function/1(FaultIDs)
  Mux1/1 -> MATLAB Function/5(unused)
  MATLAB Function/1(y) -> Data Type Conversion3/1
  Data Type Conversion/1 -> Mux12/1
  Data Type Conversion1/1 -> Mux12/2
  Data Type Conversion2/1 -> Mux12/3
  Data Type Conversion3/1 -> Mux12/4
  Mux12/1 -> logOut/1

== system QuadModelv/Motor FaultModel ==
  Battery Model Bus : Inport
  Bus Selector : BusSelector  OutputSignals=PWMOut
  MotorFault : QuadModelLib/MotorFault  FaultParamStruct=MotorFault1  ComParamVect=FaultParamAPI
  Motor_Fun : Subsystem
  MotorRads : Outport  VectorParamsAs1DForOutWhenUnconnected=off
  wires:
  Battery Model Bus/1 -> Bus Selector/1
  [FaultIn] -> MotorFault/1
  Bus Selector/1 -> MotorFault/2  "<PWMOut>"
  MotorFault/1 -> Motor_Fun/1(PWMIn)
  Motor_Fun/1(PWMOut) -> MotorRads/1

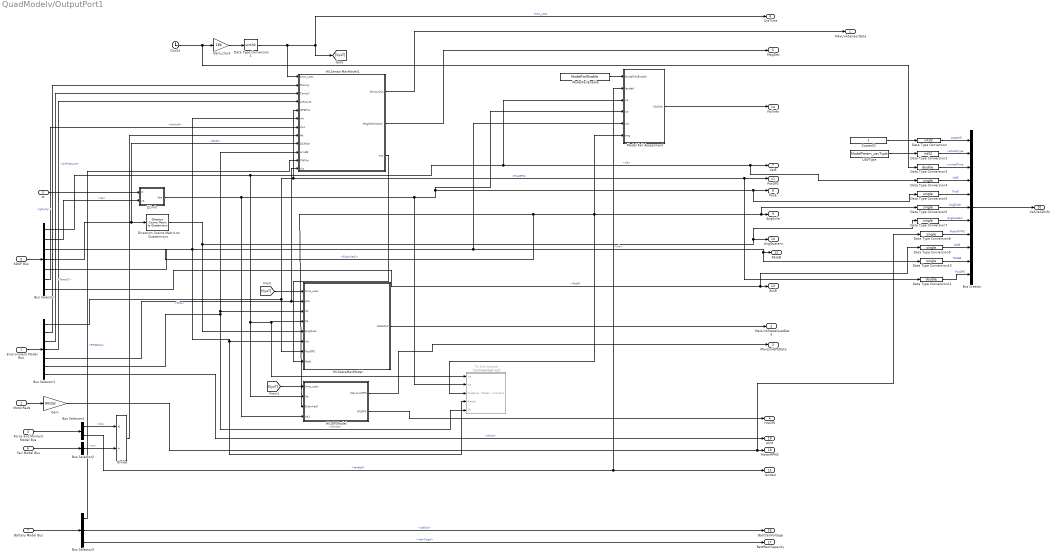
== system QuadModelv/OutputPort1 ==
  Environment Model Bus : Inport
  MotorRads : Inport  Port=2
  zt : Inport  Port=3
  Force and Moment Model Bus : Inport  Port=4
  6DOF Bus : Inport  Port=5
  Fail Model Bus : Inport  Port=6
  Battery Model Bus : Inport  Port=7
  Bus Creator : BusCreator  Inputs=11  OutDataTypeStr=Bus: MavVehileInfo
  Bus Selector : BusSelector  OutputSignals=Ve,Xe,Eular(rad),DCM,wb,dwb/dt,AccB
  Bus Selector1 : BusSelector  OutputSignals=PosGPS,gravity,TempC,AirPressure,Rho,Windb,Wind
  Bus Selector2 : BusSelector  OutputSignals=m
  Bus Selector3 : BusSelector  OutputSignals=PWMOut,cellVol,remCapa
  Bus Selector4 : BusSelector  OutputSignals=Fb,landed
  Clock1 : Clock
  CopterID : Constant
  Data Type Conversion : DataTypeConversion  OutDataTypeStr=int32  SaturateOnIntegerOverflow=off  RndMeth=Floor
  Data Type Conversion1 : DataTypeConversion  OutDataTypeStr=uint32  SaturateOnIntegerOverflow=off  RndMeth=Floor
  Data Type Conversion{4..10} (7 alike) : DataTypeConversion  OutDataTypeStr=single  SaturateOnIntegerOverflow=off  RndMeth=Floor
  Data Type Conversion11 : DataTypeConversion  OutDataTypeStr=double  SaturateOnIntegerOverflow=off  RndMeth=Floor
  Data Type Conversion2 : DataTypeConversion  OutDataTypeStr=int32  SaturateOnIntegerOverflow=off  RndMeth=Floor
  Data Type Conversion3 : DataTypeConversion  OutDataTypeStr=double  SaturateOnIntegerOverflow=off  RndMeth=Floor
  Direction Cosine Matrix to Quaternions : sharedtransform/Direction Cosine Matrix  to Quaternions  aMode=aMode  action=None  tolerance=eps(2)
      settings: SourceProductBaseCode=AE,PW,DR,MT,VE
  Divide : Product  Inputs=*/
  Gain : Gain  Gain=60/2/pi
  Gain_clock : Gain  Gain=1E6
  HILGPSModel : Subsystem
  HILSensorMavModel1 : Subsystem
  HILStateMavModel : Subsystem
  Model Fail Assessment : MATLAB Function  TreatAsAtomicUnit=on
  ModelFailEnable : Constant  Value=ModelFailEnable
  To Sim Control : Subsystem  Commented=on
  UAVType : Constant  Value=ModelParam_uavType
  ZLimit : MATLAB Function  TreatAsAtomicUnit=on
  MavLinkSensorData : Outport  VectorParamsAs1DForOutWhenUnconnected=off
  MavLinkStateQuatData : Outport  Port=2  VectorParamsAs1DForOutWhenUnconnected=off
  MavLinkGPSData : Outport  Port=3  VectorParamsAs1DForOutWhenUnconnected=off
  HILGPS : Outport  Port=4  VectorParamsAs1DForOutWhenUnconnected=off
  MagDec : Outport  Port=5  VectorParamsAs1DForOutWhenUnconnected=off
  SysTime : Outport  Port=6  VectorParamsAs1DForOutWhenUnconnected=off
  VelE : Outport  Port=7  VectorParamsAs1DForOutWhenUnconnected=off
  PosE : Outport  Port=8  VectorParamsAs1DForOutWhenUnconnected=off
  AngEuler : Outport  Port=9  VectorParamsAs1DForOutWhenUnconnected=off
  AngQuatern : Outport  Port=10  VectorParamsAs1DForOutWhenUnconnected=off
  PosGPS : Outport  Port=11  VectorParamsAs1DForOutWhenUnconnected=off
  RateB : Outport  Port=12  VectorParamsAs1DForOutWhenUnconnected=off
  AccB : Outport  Port=13  VectorParamsAs1DForOutWhenUnconnected=off
  FailInfo : Outport  Port=14  VectorParamsAs1DForOutWhenUnconnected=off
  landed : Outport  Port=15  VectorParamsAs1DForOutWhenUnconnected=off
  BattCellVoltage : Outport  Port=16  VectorParamsAs1DForOutWhenUnconnected=off
  BattRemCapacity : Outport  Port=17  VectorParamsAs1DForOutWhenUnconnected=off
  MotorRPMS : Outport  Port=18  VectorParamsAs1DForOutWhenUnconnected=off
  wind : Outport  Port=19  VectorParamsAs1DForOutWhenUnconnected=off
  Vehile3DInfo : Outport  Port=20  VectorParamsAs1DForOutWhenUnconnected=off
  wires:
  [SysT] -> HILGPSModel/1(time_usec)
  [SysT] -> HILStateMavModel/1(time_usec)
  Bus Selector/5 -> HILSensorMavModel1/6(wb), Data Type Conversion10/1, RateB/1, Model Fail Assessment/5(wb), To Sim Control/4(Rateb), HILStateMavModel/6(wb)  "<wb>"
  Bus Selector/4 -> HILSensorMavModel1/9(DCMbe), Direction Cosine Matrix to Quaternions/1  "<DCM>"
  Bus Selector/1 -> HILGPSModel/2(Ve), To Sim Control/1(Ve), HILStateMavModel/4(Ve), Model Fail Assessment/3(ve), Data Type Conversion4/1, VelE/1  "<Ve>"
  Bus Selector/6 -> HILSensorMavModel1/7(dwt)  "<dwb/dt>"
  Bus Selector/3 -> Data Type Conversion6/1, AngEuler/1, Model Fail Assessment/6(ang), To Sim Control/3(AngEuler), HILGPSModel/3(Eular(rad))  "<Eular(rad)>"
  Clock1/1 -> Data Type Conversion3/1, Gain_clock/1
  Data Type Conversion1/1 -> HILSensorMavModel1/1(time_usec), SysTime/1, [SysT]  "time_usec"
  Gain_clock/1 -> Data Type Conversion1/1
  6DOF Bus/1 -> Bus Selector/1
  zt/1 -> ZLimit/1(zt)
  Bus Selector/2 -> ZLimit/2(xe)  "<Xe>"
  Environment Model Bus/1 -> Bus Selector1/1
  Bus Selector1/1 -> HILStateMavModel/7(PosGPS), HILSensorMavModel1/5(GPSPos), Data Type Conversion11/1, PosGPS/1  "<PosGPS>"
  Bus Selector1/2 -> HILSensorMavModel1/2(Gravity)  "<gravity>"
  Bus Selector1/3 -> HILSensorMavModel1/3(TempC)  "<TempC>"
  Bus Selector1/4 -> HILSensorMavModel1/4(pressure)  "<AirPressure>"
  Bus Selector1/5 -> HILSensorMavModel1/12(rho), HILStateMavModel/2(pho)  "<Rho>"
  Bus Selector1/6 -> HILSensorMavModel1/10(windB), HILStateMavModel/3(Vb), To Sim Control/5(Vb)  "<Windb>"
  Bus Selector2/1 -> Divide/2  "<m>"
  Bus Selector4/1 -> Divide/1  "<Fb>"
  Force and Moment Model Bus/1 -> Bus Selector4/1
  Fail Model Bus/1 -> Bus Selector2/1
  Bus Selector4/2 -> landed/1, Model Fail Assessment/2(landed)  "<landed>"
  Battery Model Bus/1 -> Bus Selector3/1
  Bus Selector3/2 -> BattCellVoltage/1  "<cellVol>"
  Bus Selector3/3 -> BattRemCapacity/1  "<remCapa>"
  Bus Selector3/1 -> HILSensorMavModel1/11(PWMin)  "<PWMOut>"
  Bus Selector1/7 -> wind/1  "<Wind>"
  MotorRads/1 -> Gain/1
  HILSensorMavModel1/1(SensorOut) -> MavLinkSensorData/1
  HILSensorMavModel1/2(MagDeclination) -> MagDec/1
  Model Fail Assessment/1(FailInfo) -> FailInfo/1
  ZLimit/1(Xee) -> HILGPSModel/4(Xe1), Data Type Conversion5/1, PosE/1, Model Fail Assessment/4(xe), To Sim Control/2(Xe)
  Direction Cosine Matrix to Quaternions/1 -> Data Type Conversion7/1, AngQuatern/1, HILStateMavModel/5(AngQuat)
  Divide/1 -> HILSensorMavModel1/8(Ab)
  HILStateMavModel/1(stateOut) -> MavLinkStateQuatData/1
  HILGPSModel/1(MavLinkGPS) -> MavLinkGPSData/1
  HILGPSModel/2(HILGPS) -> HILGPS/1
  Gain/1 -> Data Type Conversion8/1, MotorRPMS/1
  Bus Selector/7 -> Data Type Conversion9/1, AccB/1  "<AccB>"
  CopterID/1 -> Data Type Conversion/1
  Data Type Conversion/1 -> Bus Creator/1  "copterID"
  Data Type Conversion2/1 -> Bus Creator/2  "vehicleType"
  UAVType/1 -> Data Type Conversion2/1
  Data Type Conversion3/1 -> Bus Creator/3  "runnedTime"
  Data Type Conversion4/1 -> Bus Creator/4  "VelE"
  Data Type Conversion5/1 -> Bus Creator/5  "PosE"
  Data Type Conversion6/1 -> Bus Creator/6  "AngEuler"
  Data Type Conversion7/1 -> Bus Creator/7  "AngQuatern"
  Data Type Conversion8/1 -> Bus Creator/8  "MotorRPMS"
  Data Type Conversion9/1 -> Bus Creator/9  "AccB"
  Data Type Conversion10/1 -> Bus Creator/10  "RateB"
  Data Type Conversion11/1 -> Bus Creator/11  "PosGPS"
  HILSensorMavModel1/3(acc) -> HILStateMavModel/8(Accb)
  ModelFailEnable/1 -> Model Fail Assessment/1(ModelFailEnable)
  Bus Creator/1 -> Vehile3DInfo/1

== system QuadModelv/Prop FaultModel ==
  MotorRadsin : Inport
  PropFault : QuadModelLib/PropFault  FaultParamStruct=PropFault  ComParamVect=FaultParamAPI
  MotorRads : Outport  VectorParamsAs1DForOutWhenUnconnected=off
  wires:
  PropFault/1 -> MotorRads/1
  [FaultIn] -> PropFault/1
  MotorRadsin/1 -> PropFault/2

== system QuadModelv/Force and Moment Model/Propeller Model ==
  uavType : Inport
  MotorRads : Inport  Port=2
  uavR : Inport  Port=3
  uavDearo : Inport  Port=4
  Cm : Inport  Port=5
  Ct : Inport  Port=6
  Jm : Inport  Port=7
  wb : Inport  Port=8
  Vb : Inport  Port=9
  Cd : Inport  Port=10
  Car : Subsystem  TreatAsAtomicUnit=on
  If : If  IfExpression=u1 >= 50
  Multicopter : Subsystem  TreatAsAtomicUnit=on
  Switch : Switch  Threshold=50  SaturateOnIntegerOverflow=off  InputSameDT=off
  Switch1 : Switch  Threshold=50  SaturateOnIntegerOverflow=off  InputSameDT=off
  Terminator : Terminator
  Terminator1 : Terminator
  Fb : Outport  VectorParamsAs1DForOutWhenUnconnected=off
  Mb : Outport  Port=2  VectorParamsAs1DForOutWhenUnconnected=off
  wires:
  Vb/1 -> Terminator/1
  Cd/1 -> Terminator1/1
  uavType/1 -> If/1, Switch/2, Switch1/2, Multicopter/1(uavType)
  Switch/1 -> Fb/1
  Switch1/1 -> Mb/1
  If/2 -> Multicopter/Action
  If/1 -> Car/Action
  Car/1(Fb) -> Switch/1
  Multicopter/1(Fb) -> Switch/3
  Car/2(Mb) -> Switch1/1
  Multicopter/2(Mb) -> Switch1/3
  MotorRads/1 -> Car/1(MotorRads), Multicopter/2(MotorRads)
  uavDearo/1 -> Multicopter/4(uavDearo)
  Cm/1 -> Multicopter/5(Cm)
  Ct/1 -> Multicopter/6(Ct)
  Jm/1 -> Multicopter/7(Jm)
  wb/1 -> Multicopter/8(wb)
  uavR/1 -> Multicopter/3(uavR)

== system QuadModelv/Motor FaultModel/Motor_Fun ==
  PWMIn : Inport
  Demux : Demux  Outputs=8
  ModelInit_RPM : Constant  Value=ModelInit_RPM
  ModelParam.motorCr : Constant  Value=ModelParam_motorCr
  ModelParam.motorT : Constant  Value=ModelParam_motorT
  ModelParam.motorWb : Constant  Value=ModelParam_motorWb
  MotorNonlinearDynamic1 : Subsystem  TreatAsAtomicUnit=on
  MotorNonlinearDynamic2 : Subsystem  TreatAsAtomicUnit=on
  MotorNonlinearDynamic3 : Subsystem  TreatAsAtomicUnit=on
  MotorNonlinearDynamic4 : Subsystem  TreatAsAtomicUnit=on
  MotorNonlinearDynamic5 : Subsystem  TreatAsAtomicUnit=on
  MotorNonlinearDynamic6 : Subsystem  TreatAsAtomicUnit=on
  MotorNonlinearDynamic7 : Subsystem  TreatAsAtomicUnit=on
  MotorNonlinearDynamic8 : Subsystem  TreatAsAtomicUnit=on
  Mux : Mux  Inputs=8
  PWMOut : Outport
  wires:
  Demux/8 -> MotorNonlinearDynamic8/5(PWM)
  ModelParam.motorWb/1 -> MotorNonlinearDynamic1/1(Wb), MotorNonlinearDynamic2/1(Wb), MotorNonlinearDynamic3/1(Wb), MotorNonlinearDynamic4/1(Wb), MotorNonlinearDynamic5/1(Wb), MotorNonlinearDynamic6/1(Wb), MotorNonlinearDynamic8/1(Wb), MotorNonlinearDynamic7/1(Wb)
  ModelParam.motorCr/1 -> MotorNonlinearDynamic1/2(Cr), MotorNonlinearDynamic2/2(Cr), MotorNonlinearDynamic3/2(Cr), MotorNonlinearDynamic4/2(Cr), MotorNonlinearDynamic5/2(Cr), MotorNonlinearDynamic6/2(Cr), MotorNonlinearDynamic8/2(Cr), MotorNonlinearDynamic7/2(Cr)
  ModelInit_RPM/1 -> MotorNonlinearDynamic2/4(ModelInit_RPM), MotorNonlinearDynamic3/4(ModelInit_RPM), MotorNonlinearDynamic4/4(ModelInit_RPM), MotorNonlinearDynamic5/4(ModelInit_RPM), MotorNonlinearDynamic6/4(ModelInit_RPM), MotorNonlinearDynamic8/4(ModelInit_RPM), MotorNonlinearDynamic7/4(ModelInit_RPM), MotorNonlinearDynamic1/4(ModelInit_RPM)
  MotorNonlinearDynamic7/1(radW) -> Mux/7
  Demux/4 -> MotorNonlinearDynamic4/5(PWM)
  Demux/7 -> MotorNonlinearDynamic7/5(PWM)
  MotorNonlinearDynamic2/1(radW) -> Mux/2
  ModelParam.motorT/1 -> MotorNonlinearDynamic2/3(motorT), MotorNonlinearDynamic3/3(motorT), MotorNonlinearDynamic4/3(motorT), MotorNonlinearDynamic5/3(motorT), MotorNonlinearDynamic6/3(motorT), MotorNonlinearDynamic8/3(motorT), MotorNonlinearDynamic7/3(motorT), MotorNonlinearDynamic1/3(motorT)
  MotorNonlinearDynamic1/1(radW) -> Mux/1
  Demux/6 -> MotorNonlinearDynamic6/5(PWM)
  MotorNonlinearDynamic6/1(radW) -> Mux/6
  MotorNonlinearDynamic5/1(radW) -> Mux/5
  Demux/1 -> MotorNonlinearDynamic1/5(PWM)
  MotorNonlinearDynamic8/1(radW) -> Mux/8
  Demux/3 -> MotorNonlinearDynamic3/5(PWM)
  MotorNonlinearDynamic4/1(radW) -> Mux/4
  Demux/5 -> MotorNonlinearDynamic5/5(PWM)
  Demux/2 -> MotorNonlinearDynamic2/5(PWM)
  MotorNonlinearDynamic3/1(radW) -> Mux/3
  PWMIn/1 -> Demux/1
  Mux/1 -> PWMOut/1

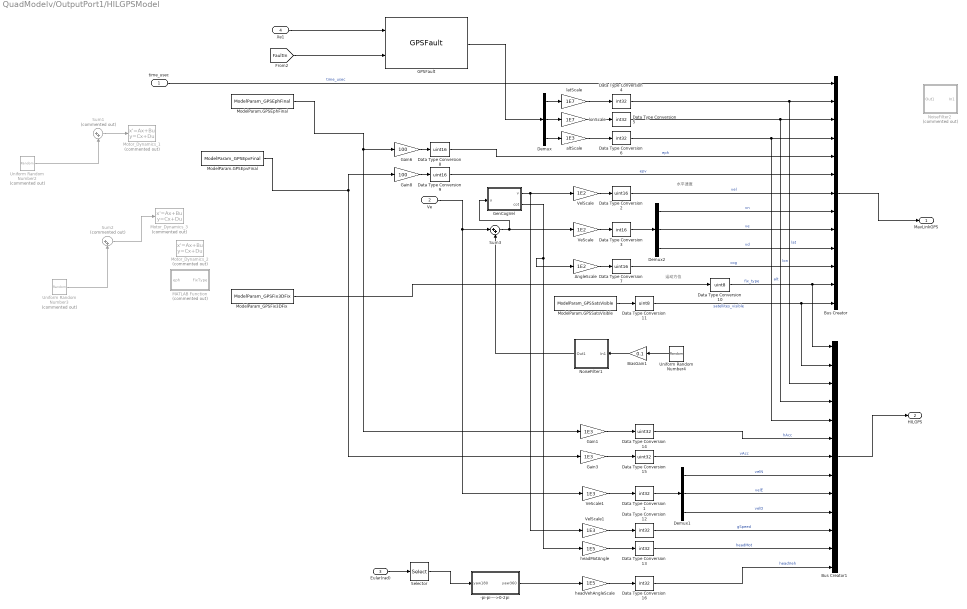
== system QuadModelv/OutputPort1/HILGPSModel ==
  note: 水平速度
  note: 运动方位
  time_usec : Inport
  Ve : Inport  Port=2
  Eular(rad) : Inport  Port=3
  Xe1 : Inport  Port=4
  -pi-pi---->0-2pi : MATLAB Function  TreatAsAtomicUnit=on
  AngleScale : Gain  Gain=1E2
  BiasGain1 : Gain  Gain=0.1
  Bus Creator : BusCreator  Inputs=13  OutDataTypeStr=Bus: MavLinkGPS  NonVirtualBus=on
  Bus Creator1 : BusCreator  Inputs=13  OutDataTypeStr=Bus: HILGPS  NonVirtualBus=on
  Data Type Conversion{1,4..6,12..13,16} (7 alike) : DataTypeConversion  OutDataTypeStr=int32  RndMeth=Round  SaturateOnIntegerOverflow=off
  Data Type Conversion10 : DataTypeConversion  OutDataTypeStr=uint8  RndMeth=Round  SaturateOnIntegerOverflow=off
  Data Type Conversion11 : DataTypeConversion  OutDataTypeStr=uint8  RndMeth=Round  SaturateOnIntegerOverflow=off
  Data Type Conversion14 : DataTypeConversion  OutDataTypeStr=uint32  RndMeth=Round  SaturateOnIntegerOverflow=off
  Data Type Conversion15 : DataTypeConversion  OutDataTypeStr=uint32  RndMeth=Round  SaturateOnIntegerOverflow=off
  Data Type Conversion{2,7..9} (4 alike) : DataTypeConversion  OutDataTypeStr=uint16  RndMeth=Round  SaturateOnIntegerOverflow=off
  Data Type Conversion3 : DataTypeConversion  OutDataTypeStr=int16  RndMeth=Round  SaturateOnIntegerOverflow=off
  Demux : Demux  Outputs=3
  Demux1 : Demux  Outputs=3
  Demux2 : Demux  Outputs=3
  GPSFault : QuadModelLib/GPSFault  FaultParamStruct=SensorFault
  Gain1 : Gain  Gain=1E3
  Gain3 : Gain  Gain=1E3
  Gain6 : Gain  Gain=100
  Gain8 : Gain  Gain=100
  GenCogVel : MATLAB Function  TreatAsAtomicUnit=on
  MATLAB Function : MATLAB Function  Commented=on  TreatAsAtomicUnit=on
  ModelParam.GPSEphFinal : Constant  Value=ModelParam_GPSEphFinal
  ModelParam.GPSEpvFinal : Constant  Value=ModelParam_GPSEpvFinal
  ModelParam.GPSSatsVisible : Constant  Value=ModelParam_GPSSatsVisible
  ModelParam_GPSFix3DFix : Constant  Value=ModelParam_GPSFix3DFix
  Motor_Dynamics_1 : StateSpace  Commented=on  A=-1/0.2  C=1/0.2  D=0  InitialCondition=20*0.2
  Motor_Dynamics_2 : StateSpace  Commented=on  A=-1/ModelParam_GPSEpvTimeConstant  C=1/ModelParam_GPSEpvTimeConstant  D=0  InitialCondition=ModelParam_GPSEpvInitial*ModelParam_GPSEpvTimeConstant
  Motor_Dynamics_3 : StateSpace  Commented=on  A=-1/0.2  C=1/0.2  D=0  InitialCondition=20*0.2
  NoiseFilter1 : Subsystem
  NoiseFilter2 : Subsystem  Commented=on
  Selector : Selector  InputPortWidth=3  IndexOptions=Index vector (dialog)  Indices=[3]  OutputSizes=1
  Sum1 : Sum  Commented=on  Inputs=|++
  Sum2 : Sum  Commented=on  Inputs=|++
  Sum3 : Sum  Inputs=|++
  Uniform Random Number2 : UniformRandomNumber  Commented=on  Minimum=-0.01  Maximum=0.01  Seed=4345454  SampleTime=ModelParam_noiseGPSSampTime
  Uniform Random Number3 : UniformRandomNumber  Commented=on  Seed=3244333  SampleTime=ModelParam_noiseGPSSampTime
  Uniform Random Number4 : UniformRandomNumber  Minimum=[-1,-1,-2]  Maximum=[1,1,2]  Seed=[5445,45433,33433]  SampleTime=ModelParam_noiseGPSSampTime
  VeScale : Gain  Gain=1E2
  VeScale1 : Gain  Gain=1E3
  VelScale : Gain  Gain=1E2
  VelScale1 : Gain  Gain=1E3
  altScale : Gain  Gain=1E3
  headMotAngle : Gain  Gain=1E5
  headVehAngleScale : Gain  Gain=1E5
  latScale : Gain  Gain=1E7
  lonScale : Gain  Gain=1E7
  MavLinkGPS : Outport  VectorParamsAs1DForOutWhenUnconnected=off
  HILGPS : Outport  Port=2  VectorParamsAs1DForOutWhenUnconnected=off
  wires:
  Data Type Conversion16/1 -> Bus Creator1/13  "headVeh"
  headVehAngleScale/1 -> Data Type Conversion16/1
  Data Type Conversion13/1 -> Bus Creator1/12  "headMot"
  Data Type Conversion12/1 -> Bus Creator1/11  "gSpeed"
  Demux1/3 -> Bus Creator1/10  "velD"
  Demux1/2 -> Bus Creator1/9  "velE"
  Demux1/1 -> Bus Creator1/8  "velN"
  Data Type Conversion1/1 -> Demux1/1
  headMotAngle/1 -> Data Type Conversion13/1
  Data Type Conversion15/1 -> Bus Creator1/7  "vAcc"
  Data Type Conversion14/1 -> Bus Creator1/6  "hAcc"
  Gain3/1 -> Data Type Conversion15/1
  Gain1/1 -> Data Type Conversion14/1
  VeScale1/1 -> Data Type Conversion1/1
  VelScale1/1 -> Data Type Conversion12/1
  Data Type Conversion8/1 -> Bus Creator/5  "eph"
  Gain8/1 -> Data Type Conversion9/1
  Gain6/1 -> Data Type Conversion8/1
  Data Type Conversion9/1 -> Bus Creator/6  "epv"
  time_usec/1 -> Bus Creator/1  "time_usec"
  latScale/1 -> Data Type Conversion4/1
  lonScale/1 -> Data Type Conversion5/1
  altScale/1 -> Data Type Conversion6/1
  Data Type Conversion4/1 -> Bus Creator/2, Bus Creator1/3  "lat"
  Data Type Conversion5/1 -> Bus Creator/3, Bus Creator1/4  "lon"
  Data Type Conversion6/1 -> Bus Creator/4, Bus Creator1/5  "alt"
  Demux2/1 -> Bus Creator/8  "vn"
  Demux2/2 -> Bus Creator/9  "ve"
  Demux2/3 -> Bus Creator/10  "vd"
  VeScale/1 -> Data Type Conversion3/1
  Data Type Conversion3/1 -> Demux2/1
  VelScale/1 -> Data Type Conversion2/1
  Data Type Conversion2/1 -> Bus Creator/7  "vel"
  AngleScale/1 -> Data Type Conversion7/1
  Data Type Conversion7/1 -> Bus Creator/11  "cog"
  Data Type Conversion11/1 -> Bus Creator/13, Bus Creator1/2  "satellites_visible"
  Data Type Conversion10/1 -> Bus Creator/12, Bus Creator1/1  "fix_type"
  ModelParam.GPSSatsVisible/1 -> Data Type Conversion11/1
  Demux/1 -> latScale/1
  Demux/2 -> lonScale/1
  Demux/3 -> altScale/1
  ModelParam.GPSEphFinal/1 -> Gain1/1, Gain6/1
  Sum2/1 -> Motor_Dynamics_3/1
  ModelParam_GPSFix3DFix/1 -> Data Type Conversion10/1
  Ve/1 -> VeScale1/1, Sum3/1
  GenCogVel/1(v) -> VelScale/1, VelScale1/1
  Eular(rad)/1 -> Selector/1
  Bus Creator/1 -> MavLinkGPS/1
  Bus Creator1/1 -> HILGPS/1
  -pi-pi---->0-2pi/1(yaw360) -> headVehAngleScale/1
  Selector/1 -> -pi-pi---->0-2pi/1(yaw180)
  BiasGain1/1 -> NoiseFilter1/1(In1)
  Uniform Random Number4/1 -> BiasGain1/1
  GenCogVel/2(cot) -> AngleScale/1, headMotAngle/1
  Sum1/1 -> Motor_Dynamics_1/1
  Uniform Random Number2/1 -> Sum1/2
  Uniform Random Number3/1 -> Sum2/2
  ModelParam.GPSEpvFinal/1 -> Gain8/1, Gain3/1
  Sum3/1 -> GenCogVel/1(u), VeScale/1
  NoiseFilter1/1(Out1) -> Sum3/2
  [FaultIn] -> GPSFault/2
  Xe1/1 -> GPSFault/1
  GPSFault/1 -> Demux/1

== system QuadModelv/OutputPort1/HILSensorMavModel1 ==
  time_usec : Inport
  Gravity : Inport  Port=2
  TempC : Inport  Port=3
  pressure : Inport  Port=4
  GPSPos : Inport  Port=5
  wb : Inport  Port=6
  dwt : Inport  Port=7
  Ab : Inport  Port=8
  DCMbe : Inport  Port=9
  windB : Inport  Port=10
  PWMin : Inport  Port=11
  rho : Inport  Port=12
  Subsystem : Subsystem
  SensorOut : Outport  VectorParamsAs1DForOutWhenUnconnected=off
  MagDeclination : Outport  Port=2  VectorParamsAs1DForOutWhenUnconnected=off
  acc : Outport  Port=3  VectorParamsAs1DForOutWhenUnconnected=off
  wires:
  pressure/1 -> Subsystem/1(pressure)
  windB/1 -> Subsystem/2(windB)
  rho/1 -> Subsystem/3(rho)
  TempC/1 -> Subsystem/4(TempC)
  GPSPos/1 -> Subsystem/5(GPSPos)
  Ab/1 -> Subsystem/6(Ab)
  wb/1 -> Subsystem/7(wb)
  dwt/1 -> Subsystem/8(dwt)
  DCMbe/1 -> Subsystem/9(DCMbe)
  Subsystem/1(SensorOut) -> SensorOut/1
  Subsystem/2(MagDeclination) -> MagDeclination/1
  Subsystem/3(acc) -> acc/1
  PWMin/1 -> Subsystem/10(PWMin)
  Gravity/1 -> Subsystem/12(Gravity)
  time_usec/1 -> Subsystem/11(time_usec)  "time_usec"
